simulink model "Polynomial_Solver"  (R2018b)
settings: Solver=FixedStepAuto  StartTime=0.0  StopTime=10.0  RelTol=1e-3
settings Model: Creator=sulaymon.eshkabilov  LastModifiedBy=sulaymon.eshkabilov
settings SFSimCC: SimUseLocalCustomCode=off
settings RTWCC: RTWUseLocalCustomCode=off
settings CodeAppCC: StateflowObjectComments=on

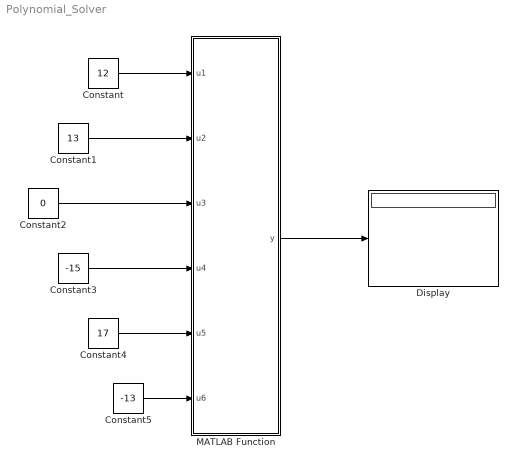
== system Polynomial_Solver ==
  Constant : Constant  Value=12
  Constant1 : Constant  Value=13
  Constant2 : Constant  Value=0
  Constant3 : Constant  Value=-15
  Constant4 : Constant  Value=17
  Constant5 : Constant  Value=-13
  Display : Display
      settings: Decimation=9
  MATLAB Function : MATLAB Function  TreatAsAtomicUnit=on
  wires:
  Constant/1 -> MATLAB Function/1(u1)
  Constant1/1 -> MATLAB Function/2(u2)
  Constant2/1 -> MATLAB Function/3(u3)
  Constant3/1 -> MATLAB Function/4(u4)
  Constant4/1 -> MATLAB Function/5(u5)
  Constant5/1 -> MATLAB Function/6(u6)
  MATLAB Function/1(y) -> Display/1

== matlab function Polynomial_Solver/MATLAB Function ==
  data: u1 input; y output size=5; u2 input; u3 input; u4 input; u5 input; u6 input
function y  = fcn(u1, u2, u3, u4, u5, u6)
y = roots([u1, u2, u3, u4, u5, u6]);
